simulink model "sf_call_pointer"  (R2021a)
settings: Solver=FixedStepDiscrete  StartTime=0.0  StopTime=10.0  RelTol=1e-3
CloseFcn:
  | clear all
  | try
  | rmdir slprj\ s
  | catch
  | end
  | try
  | folder_name = [bdroot '*'];
  | rmdir(folder_name,'s')
  | catch
  | end
  | try
  | file_temp_name = [bdroot '.slxc'];
  | delete(file_temp_name)
  | %%delete *.mexw64
  | catch
  | end
  | clear folder_name file_temp_name
settings Model: Creator=jetson  LastModifiedBy=jetson
settings DataIOCC: SaveOutput=off  SignalLogging=off  DSMLogging=off  SaveTime=off  ReturnWorkspaceOutputs=off
settings OptimizationCC: DefaultParameterBehavior=Inlined  EnhancedBackFolding=on  PassReuseOutputArgsAs=Individual arguments  ZeroExternalMemoryAtStartup=off  ZeroInternalMemoryAtStartup=off  OptimizeBlockOrder=speed  DifferentSizesBufferReuse=on  OptimizationCustomize=off  EfficientTunableParamExpr=on
settings DebuggingCC: ParameterTunabilityLossMsg=error
settings SFSimCC: MATLABDynamicMemAlloc=off
settings RTWCC: SystemTargetFile=ert.tlc  GenCodeOnly=on  TemplateMakefile=ert_default_tmf  GenerateReport=on  CustomSource=data_array.c  IncludeHyperlinkInReport=on  LaunchReport=on  GenerateTraceInfo=on
settings CodeAppCC: ForceParamTrailComments=on  IgnoreCustomStorageClasses=off  OperatorAnnotations=on  SimulinkDataObjDesc=on  SFDataObjDesc=on  InsertBlockDesc=on
settings ERTTargetCC: TargetLangStandard=C99 (ISO)  GenerateSampleERTMain=on  InlinedParameterPlacement=NonHierarchical  ERTCustomFileTemplate=example_file_process.tlc

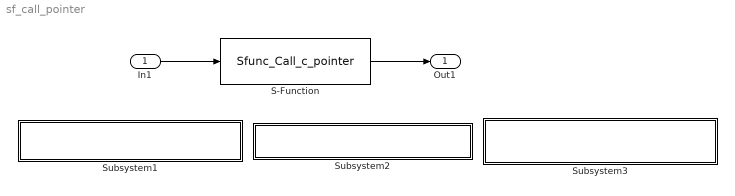
== system sf_call_pointer ==
  In1 : Inport  PortDimensions=100
      settings: AttributesFormatString=Data Type : %<OutDataTypeStr>
  S-Function : S-Function  FunctionName=Sfunc_Call_c_pointer  SFunctionDeploymentMode=off  EnableBusSupport=off
  Subsystem1 : Subsystem
      settings: OpenFcn=mex -IC_Files ./Sfunction_TLC/Sfunc_Call_c_pointer.c ./C_Files/data_array.c -outdir ./Sfunction_TLC/
      mask Display:
      | color('r')
      | disp('double click will compile Sfunc_Call_c_pointer.c')
  Subsystem2 : Subsystem
      settings: OpenFcn=edit Sfunc_Call_c_pointer.c
      mask Display:
      | color('r')
      | disp('double click will open Sfunc_Call_c_pointer.c')
  Subsystem3 : Subsystem
      settings: OpenFcn=edit Sfunc_Call_c_pointer.tlc
      mask Display:
      | color('r')
      | disp('double click will compile Sfunc_Call_c_pointer.tlc')
  Out1 : Outport
      settings: AttributesFormatString=Data Type : %<OutDataTypeStr>
  wires:
  In1/1 -> S-Function/1
  S-Function/1 -> Out1/1

== system sf_call_pointer/Subsystem1 ==

== system sf_call_pointer/Subsystem2 ==

== system sf_call_pointer/Subsystem3 ==
